simulink model "PMSM_DemoBackup"  (R2020a)
settings: Solver=FixedStepDiscrete  StartTime=0.0  StopTime=Inf  FixedStep=1000e-6  RelTol=1e-3  EnableMultiTasking=on
PreLoadFcn:
  | run('PMSM_Demo_ini.m');
PostLoadFcn:
  | , if any(exist('dsrtsu_mdlpostloadfcn', 'file') ~= 0), dsrtsu_mdlpostloadfcn('Execute', bdroot); end,
InitFcn:
  | , if any(exist('rtifpga_mdlclblib', 'file') ~= 0), rtifpga_mdlclblib('Init', bdroot); end,
undefined symbols (not defined in the file): clock, Const_Id_Fieldweakening, Const_Ld_Stator, Const_Lq_Stator, Const_PolePairs, Const_Psi, Newton, PMSM_Ctrl_Ctrl_mode_SW, PMSM_Ctrl_fRS_Set, PMSM_Ctrl_i_d_Set, PMSM_Ctrl_i_d_Stroke, PMSM_Ctrl_i_q_Set, PMSM_Ctrl_i_q_Stroke, PMSM_Ctrl_Ki_id, PMSM_Ctrl_Ki_iq, PMSM_Ctrl_Ki_n, PMSM_Ctrl_Kp_id, PMSM_Ctrl_Kp_iq, PMSM_Ctrl_Kp_n, PMSM_Ctrl_Limit_iq, PMSM_Ctrl_load_torque, PMSM_Ctrl_n_Limit, PMSM_Ctrl_n_Set, PMSM_Ctrl_n_Stroke, PMSM_Ctrl_Pos_Src, PMSM_Ctrl_TF_Id, PMSM_Ctrl_TF_Iq, PMSM_Ctrl_TF_n, PMSM_Ctrl_theta_offset, PMSM_Ctrl_v_d_Set, PMSM_Ctrl_V_DCLink_Limit, PMSM_Ctrl_v_q_Set, PMSM_Ctrl_Vel_Src, Raphson, rpm_to_rad, s, SW_Fieldweakening, T_PWM
libraries: simulink x37, rti1202lib_adc_class1 x8, dsextras x4, rtiemclib x4, rti1202lib_dio_class1 x3, ASM_ElectricComponents_lib x2, ASM_Utils_lib x1, rti1202lib_base x1
(part 1 of 4)
settings Model: RTICANMMDATA=struct('GeneralSetupData',struct('modelroot','D:\PMSM_ControlDesk','generalsettings',struct('filesettings',struct('destfolder',struct('Name','RTICANMM_FILES','Check',1),'buildfolder',struct('Name','.','Check',1),'AbsDestfolder',struct('Name','D:\PMSM_ControlDesk\RTICANMM_FILES'),'AbsBuildfolder',struct('Name','D:\PMSM_ControlDesk'))),'options',struct('addpaths',1,'rmpaths',1,'addtrcexclusion',true,'cannavigator',struct('checkmonitoring',0),'show_usrtrc',0,'use_usrtrc',0),'advanced',struct('options',ones(1,100)),'MPSetup',{{}},'RTI',struct('Type','RTI1202','Ver','7.15','Date','02-Nov-2020'),'modelname','PMSM_DemoBackup','block','PMSM_DemoBackup'))  RTILINMMDATA=struct('GeneralSetupData',[])  DSRTSU_INTERNAL_RTI_VER=570  DSRTSU_INTERNAL_RTI_TYPE=rti1202  DSRTSU_INTERNAL_RTIFPGA=170  Creator=JesseL  LastModifiedBy=PC2
settings DataIOCC: LimitDataPoints=on  SaveFormat=Array  SignalLoggingSaveFormat=ModelDataLogs  ReturnWorkspaceOutputs=off
settings OptimizationCC: BlockReduction=off  ConditionallyExecuteInputs=off  OptimizeBlockIOStorage=off  BufferReuse=off  GlobalBufferReuse=off  ExpressionFolding=off  ExpressionDepthLimit=2147483647  LocalBlockOutputs=off  InitFltsAndDblsToZero=on  LifeSpan=inf  OptimizeDataStoreBuffers=off  BusAssignmentInplaceUpdate=off
settings DebuggingCC: SaveWithParameterizedLinksMsg=none  UnderspecifiedInitializationDetection=Classic  MergeDetectMultiDrivingBlocksExec=none  SignalResolutionControl=TryResolveAllWithWarning  SolverPrmCheckMsg=warning  MultiTaskDSMMsg=warning  MultiTaskCondExecSysMsg=none  AllowSymbolicDim=off  StateNameClashWarn=warning  SFUnexpectedBacktrackingDiag=warning  SFNoUnconditionalDefaultTransitionDiag=warning  SFExecutionAtInitializationDiag=none  ArithmeticOperatorsInVariantConditions=warning
settings HardwareCC: ProdBitPerPointer=32  ProdBitPerSizeT=32  ProdBitPerPtrDiffT=32  ProdLargestAtomicInteger=Integer  ProdEndianess=BigEndian  ProdWordSize=32  ProdHWDeviceType=Custom Processor->Custom  TargetIntDivRoundTo=Zero  TargetEndianess=BigEndian  TargetHWDeviceType=Custom Processor->Custom
settings ModelReferenceCC: PropagateSignalLabelsOutOfModel=off
settings SFSimCC: SimUseLocalCustomCode=off  MATLABDynamicMemAlloc=off  CustomCodeUndefinedFunction=UseInterfaceOnly
settings RTWCC: Description=dSPACE DS1202 Hardware Platform  SystemTargetFile=rti1202.tlc  MakeCommand=make_rti  TemplateMakefile=rti1202.tmf  RTWUseLocalCustomCode=off
settings CodeAppCC: StateflowObjectComments=on
settings STFCustomTargetCC: ParMdlRefBuildCompliant=on  SystemTargetFile=rti1202.tlc
settings GRTTargetCC: TargetLangStandard=C89/C90 (ANSI)  CompOptLevelCompliant=off  ConcurrentExecutionCompliant=off  CombineOutputUpdateFcns=off  MatFileLogging=off  CPPClassGenCompliant=off  UseToolchainInfoCompliant=off  ExtModeMexFile=noextcomm
settings ConfigComp: CovMetricSettings=dw  CovHtmlReporting=on  CovSaveCumulativeToWorkspaceVar=on  CovSaveSingleToWorkspaceVar=on  CovExternalEMLEnable=off

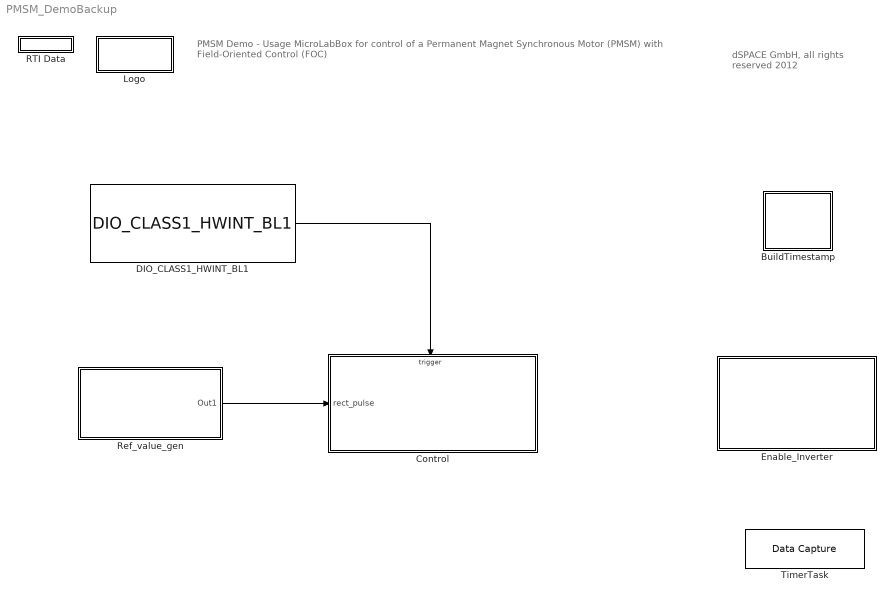
== system PMSM_DemoBackup ==
  note: PMSM Demo - Usage MicroLabBox for control
      | of a Permanent Magnet Synchronous Motor (PMSM)
      | with Field-Oriented Control (FOC)
  note: dSPACE GmbH,
      | all rights reserved 2012
  BuildTimestamp : Subsystem
  Control : Subsystem
  DIO_CLASS1_HWINT_BL1 : rti1202lib_dio_class1/DIO_CLASS1_HWINT_BL1  DSProperties=struct('RTI',struct('Version',uint32(2),'BlockType',struct('isSLSource',uint8(1),'isSLSink',uint8(0),'isHWSource',uint8(0),'isHWSink',uint8(0),'isSetup',uint8(0),'isInline',uint8(1),'isNonInline',uint8(0),'isInterrupt',uint8(1),'isChannelwise',uint8(0)),'IOBoardType',{{'DS120X','STD','DIOC1'}},'UnitType','DSTASKTOOL','Identifier','HWINT','DialogType','ML','BlockSet','NONE','SlaveProcessor','NONE'))  RTIBlockInterface=struct('OutputPortsActive',1,'OutputPortsWidth',int32(1),'OutputPortsName',{{'Interrupt'}},'FunctionCall',uint32(0),'DialogFcn','rti120xstddioc1hwintgui','InitLevel',3,'BlockDisplay',{{['DIO CL1 HWINT\nPort: 1\nChannel: 7'],'center'}},'IconTransparency','on','BlockName',struct('Token',{{'DIO_CLASS1_HWINT_BL1'}}))  RTIBlockParameters=struct('SourceBlockListIdx',{{2,'OFF',[1 2]}},'SourceBlockIdentifier',{{'MCPWM','OFF',[]}},'InterruptTypeListIdx',{{2,'OFF',[1 2]}},'InterruptType',{{['Center position'],'OFF',[]}},'PortNo',{{1,'OFF',[]}},'ChannelNo',{{7,'OFF',[]}})  RTISFcnParameters=struct('PortNo','int16','ChannelNo','int16')  RTIBlockParaDefault=struct('SourceBlockListIdx',1,'SourceBlockIdentifier',['NOT SELECTED'],'InterruptTypeListIdx',1,'InterruptType',['NOT SELECTED'],'PortNo',-1,'ChannelNo',-1)
  Enable_Inverter : Subsystem
      mask Display: disp('Enable_Inverter')
  Logo : Subsystem  mask(dSPACE){EmptyParameter=[]}
      mask prompts: EmptyParameter "Mask Parameter 1:"
      settings: OpenFcn=;
      mask Display: image(imread('rti_mdl_dslogo.tif'));
  RTI Data : Subsystem  Tag=struct('RTIDataServer',struct('RTIDataServerVs','2','RTIModelDescription','struct(''main'',''PMSM_DemoBackup'',''sub'','''',''isMp'',0)'))  LoadFcn="if exist('rtidc'), try,  rtidc('DataHostBlockClbLoad', gcbh); catch, disp(['Warning: ''LoadFcn'' for RTI Data block failed: ' lasterr]); end, end,"  mask(RTI_DATA_HOST){}
      mask help:
      | RTI Data Block.
      | This block is used by RTI to store internal model-dependent data.
      | Please keep this block on the root level of the model. Deleting this block will result in data loss.
      |
      | NEVER DELETE OR COPY THIS BLOCK!
      settings: CopyFcn="if exist('rtidc'), try,  rtidc('DataHostBlockClbCopy', gcbh); catch, disp(['Warning: ''CopyFcn'' for RTI Data block failed: ' lasterr]); end, end,"  DeleteFcn="if exist('rtidc'), try,  rtidc('DataHostBlockClbDelete', gcbh); catch, disp(['Warning: ''DeleteFcn'' for RTI Data block failed: ' lasterr]); end, end,"  ModelCloseFcn="if exist('rtidc'), try,  rtidc('DataHostBlockClbModelClose', gcbh); catch, disp(['Warning: ''ModelCloseFcn'' for RTI Data block failed: ' lasterr]); end, end,"  PreSaveFcn="if exist('rtidc'), try,  rtidc('DataHostBlockClbPreSave', gcbh); catch, disp(['Warning: ''PreSaveFcn'' for RTI Data block failed: ' lasterr]); end, end,"  PostSaveFcn="if exist('rtidc'), try,  rtidc('DataHostBlockClbPostSave', gcbh); catch, disp(['Warning: ''PostSaveFcn'' for RTI Data block failed: ' lasterr]); end, end,"  NameChangeFcn="if exist('rtidc'), try,  rtidc('DataHostBlockClbNameChange', gcbh); catch, disp(['Warning: ''NameChangeFcn'' for RTI Data block failed: ' lasterr]); end, end,"
      mask Help:
      | RTI Data Block.
      | This block is used by RTI to store internal model-dependent data.
      | Please keep this block on the root level of the model. Deleting this block will result in data loss.
      | 
      | NEVER DELETE OR COPY THIS BLOCK!
      mask Display:
      | text(0.5, 0.5, 'RTI Data', 'HorizontalAlignment', 'center');
      | plot([1 0]);
  Ref_value_gen : Subsystem
      mask Display: disp('Generate Reference Values')
  TimerTask : dsextras/Data Capture  ServiceNumber=4  ServiceName=TimerTask_top  SampleTime=-1  XAxisLabelMode=off  XAxisLabel=sec  XAxisIncrement=1  TLCFileName=rti_data_capture  XAxisUnit=[]  IncrementSetting=[]  CustomSampleTime=[]  Reserved1=[]  Reserved2=[]  Reserved3=[]  Reserved4=[]  DSProperties=struct('RTI',struct('Version',uint32(3),'BlockType',struct('isSLSource',uint8(0),'isSLSink',uint8(0),'isHWSource',uint8(0),'isHWSink',uint8(0),'isSetup',uint8(0),'isInline',uint8(1),'isNonInline',uint8(0),'isInterrupt',uint8(0),'isChannelwise',uint8(0)),'IOBoardType','EXTRAS','UnitType','DATACAP','Identifier','DATACAP','DialogType','SL','BlockSet','NONE','SlaveProcessor','NONE'))  RTIBlockInterface=struct('OutputPortsActive',0,'OutputPortsWidth',int32(0),'InitLevel',2,'BlockDisplay',{{['Host Service #4\nTimerTask_top'],'center'}},'BlockName',struct('Token',{{['Data Capture']}}),'MaskDescription',['Places the host service code for ControlDesk in a specific task.'],'IconTransparency','off','SampleTime',{{-1}})  RTIBlockParameters=struct('ServiceNumber',{{4,'OFF',[]}},'ServiceName',{{'TimerTask_top','OFF',[]}},'SampleTime',{{-1,'OFF',[]}},'XAxisLabelMode',{{false,'OFF',[]}},'XAxisLabel',{{'sec','OFF',[]}},'XAxisIncrement',{{1,'OFF',[]}},'TLCFileName',{{'rti_data_capture','OFF',[]}})  RTISFcnParameters=struct('ServiceNumber','double','ServiceName','char','SampleTime','double','XAxisLabelMode','double','XAxisLabel','char','XAxisIncrement','double','TLCFileName','char')  RTIBlockParaDefault=struct('ServiceNumber',1,'ServiceName','ServiceName','SampleTime',-1,'XAxisLabelMode',0,'XAxisLabel','sec','XAxisIncrement',1,'TLCFileName','rti_data_capture')
  wires:
  Ref_value_gen/1(Out1) -> Control/1(rect_pulse)
  DIO_CLASS1_HWINT_BL1/1 -> Control/Trigger

== system PMSM_DemoBackup/BuildTimestamp ==
  Demux : Demux  Outputs=6
  Terminator{,1..5} (6 alike) : Terminator
  clock : Constant  Value=clock()
  wires:
  clock/1 -> Demux/1
  Demux/1 -> Terminator/1  "01_year"
  Demux/2 -> Terminator1/1  "02_month"
  Demux/3 -> Terminator2/1  "03_day"
  Demux/4 -> Terminator3/1  "04_hour"
  Demux/5 -> Terminator4/1  "05_minute"
  Demux/6 -> Terminator5/1  "06_second"

== system PMSM_DemoBackup/Control ==
  rect_pulse : Inport
  function : TriggerPort  TriggerType=function-call  VariantControl=Variant
  Control_load_machine : Subsystem
      mask Display: disp('Load machine Ctrl')
  Controller : Subsystem
  Data Capture : dsextras/Data Capture  ServiceNumber=1  ServiceName=ASYNTask  SampleTime=-1  XAxisLabelMode=off  XAxisLabel=sec  XAxisIncrement=1  TLCFileName=rti_data_capture  XAxisUnit=[]  IncrementSetting=[]  CustomSampleTime=[]  Reserved1=[]  Reserved2=[]  Reserved3=[]  Reserved4=[]  DSProperties=struct('RTI',struct('Version',uint32(3),'BlockType',struct('isSLSource',uint8(0),'isSLSink',uint8(0),'isHWSource',uint8(0),'isHWSink',uint8(0),'isSetup',uint8(0),'isInline',uint8(1),'isNonInline',uint8(0),'isInterrupt',uint8(0),'isChannelwise',uint8(0)),'IOBoardType','EXTRAS','UnitType','DATACAP','Identifier','DATACAP','DialogType','SL','BlockSet','NONE','SlaveProcessor','NONE'))  RTIBlockInterface=struct('OutputPortsActive',0,'OutputPortsWidth',int32(0),'InitLevel',2,'BlockDisplay',{{['Host Service #1\nASYNTask'],'center'}},'BlockName',struct('Token',{{['Data Capture']}}),'MaskDescription',['Places the host service code for ControlDesk in a specific task.'],'IconTransparency','off','SampleTime',{{-1}})  RTIBlockParameters=struct('ServiceNumber',{{1,'OFF',[]}},'ServiceName',{{'ASYNTask','OFF',[]}},'SampleTime',{{-1,'OFF',[]}},'XAxisLabelMode',{{false,'OFF',[]}},'XAxisLabel',{{'sec','OFF',[]}},'XAxisIncrement',{{1,'OFF',[]}},'TLCFileName',{{'rti_data_capture','OFF',[]}})  RTISFcnParameters=struct('ServiceNumber','double','ServiceName','char','SampleTime','double','XAxisLabelMode','double','XAxisLabel','char','XAxisIncrement','double','TLCFileName','char')  RTIBlockParaDefault=struct('ServiceNumber',1,'ServiceName','ServiceName','SampleTime',-1,'XAxisLabelMode',0,'XAxisLabel','sec','XAxisIncrement',1,'TLCFileName','rti_data_capture')
  Data Capture_short : dsextras/Data Capture  ServiceNumber=2  ServiceName=ASYNTask_short  SampleTime=-1  XAxisLabelMode=off  XAxisLabel=sec  XAxisIncrement=1  TLCFileName=rti_data_capture  XAxisUnit=[]  IncrementSetting=[]  CustomSampleTime=[]  Reserved1=[]  Reserved2=[]  Reserved3=[]  Reserved4=[]  DSProperties=struct('RTI',struct('Version',uint32(3),'BlockType',struct('isSLSource',uint8(0),'isSLSink',uint8(0),'isHWSource',uint8(0),'isHWSink',uint8(0),'isSetup',uint8(0),'isInline',uint8(1),'isNonInline',uint8(0),'isInterrupt',uint8(0),'isChannelwise',uint8(0)),'IOBoardType','EXTRAS','UnitType','DATACAP','Identifier','DATACAP','DialogType','SL','BlockSet','NONE','SlaveProcessor','NONE'))  RTIBlockInterface=struct('OutputPortsActive',0,'OutputPortsWidth',int32(0),'InitLevel',2,'BlockDisplay',{{['Host Service #2\nASYNTask_short'],'center'}},'BlockName',struct('Token',{{['Data Capture']}}),'MaskDescription',['Places the host service code for ControlDesk in a specific task.'],'IconTransparency','off','SampleTime',{{-1}})  RTIBlockParameters=struct('ServiceNumber',{{2,'OFF',[]}},'ServiceName',{{'ASYNTask_short','OFF',[]}},'SampleTime',{{-1,'OFF',[]}},'XAxisLabelMode',{{false,'OFF',[]}},'XAxisLabel',{{'sec','OFF',[]}},'XAxisIncrement',{{1,'OFF',[]}},'TLCFileName',{{'rti_data_capture','OFF',[]}})  RTISFcnParameters=struct('ServiceNumber','double','ServiceName','char','SampleTime','double','XAxisLabelMode','double','XAxisLabel','char','XAxisIncrement','double','TLCFileName','char')  RTIBlockParaDefault=struct('ServiceNumber',1,'ServiceName','ServiceName','SampleTime',-1,'XAxisLabelMode',0,'XAxisLabel','sec','XAxisIncrement',1,'TLCFileName','rti_data_capture')
  Input : Subsystem
  Output : Subsystem
  pmsm_ctrl_par_sig : Subsystem
      mask Display: disp('pmsm_ctrl_par_sig');
  wires:
  Controller/2(PWM_Duty[a;b;c]) -> Output/2(PWM_Duty[a,b,c])
  Input/4(n[rpm]) -> Controller/4(n[rpm])
  rect_pulse/1 -> pmsm_ctrl_par_sig/1(rect_pulse)
  Input/5(epsilon[rad]) -> Controller/5(epsilon[rad])
  Input/1(T_Sample [s]) -> Controller/1(T_Sample[s])
  Input/3(i_stator(a,b,c)[A]) -> Controller/3(i_stator[a;b;c][A])
  Controller/1(T_Sample [s]) -> Output/1(T_Sample[s])
  Input/2(V_DCLink[V]) -> Controller/2(V_DCLink[V])

== system PMSM_DemoBackup/Enable_Inverter ==
  DIO_CLASS1_BIT_OUT_BL2 : rti1202lib_dio_class1/DIO_CLASS1_BIT_OUT_BL1  DSProperties=struct('RTI',struct('Version',uint32(1),'BlockType',struct('isSLSource',uint8(0),'isSLSink',uint8(1),'isHWSource',uint8(0),'isHWSink',uint8(1),'isSetup',uint8(0),'isInline',uint8(1),'isNonInline',uint8(0),'isInterrupt',uint8(0),'isChannelwise',uint8(1)),'IOBoardType',{{'DS120X','STD','DIOC1'}},'UnitType','BIT','Identifier','BITOUT','DialogType','ML','BlockSet','NONE','SlaveProcessor','NONE'))  RTIBlockInterface=struct('InputPortsWidth',int32(1),'InputPortsActive',1,'InputPortsDataType',{{'SS_BOOLEAN'}},'InputPortsName',{{'In'}},'BlockDisplay',{{['DIO CL1 BIT OUT\nPort: 1\nChannel: 15\nNumber of channels: 1'],'center\'}},'IconTransparency','on','InitLevel',3,'DialogFcn','rti120xstddioc1bitoutgui','BlockName',struct('Token',{{'DIO_CLASS1_BIT_OUT_BL1'}}))  RTIBlockParameters=struct('PortNo',{{1,'OFF',[]}},'ChannelNo',{{15,'OFF',[]}},'ChannelNumOf',{{1,'OFF',[]}},'HighLevel',{{3,'OFF',[1 3]}},'OutputStateInit',{{zeros(1,16),'OFF',[0 1]}},'OutputStateTerm',{{zeros(1,16),'OFF',[0 1]}},'TerminationMode',{{0,'OFF',[0 1]}},'OutputStateTermValidate',{{0,'OFF',[0 1]}},'OutputStateInitSetAll',{{0,'OFF',[0 1]}},'OutputStateTermSetAll',{{0,'OFF',[0 1]}},'EnableEvent',{{0,'OFF',[0 1]}},'EventMode',{{1,'OFF',[1 3]}},'EventOnFalling',{{1,'OFF',[0 1]}},'EventOnRising',{{0,'OFF',[0 1]}},'EventDelay',{{'0','OFF',[0 1.34]}},'EventRate',{{'1','OFF',[1 256]}},'EventBuildCheck',{{false,'OFF',[]}},'TriggerLine',{{1,'OFF',[1 16]}},'EventChannelNoIdx',{{1,'OFF',[1 16]}},'TLCFileName',{{'rti120xdio_c1_bit_out','OFF',[]}})  RTISFcnParameters=struct('PortNo','int16','ChannelNo','int16','ChannelNumOf','int16','HighLevel','int16','OutputStateInit','int16','OutputStateTerm','int16','TerminationMode','int16','OutputStateTermValidate','int16','EnableEvent','int16','EventMode','int16','EventOnFalling','int16','EventOnRising','int16','EventDelay','double','EventRate','int16','TriggerLine','int16','EventChannelNoIdx','int16','TLCFileName','char')  RTIBlockParaDefault=struct('PortNo',1,'ChannelNo',1,'ChannelNumOf',1,'HighLevel',1,'OutputStateInit',zeros(1,16),'OutputStateTerm',zeros(1,16),'TerminationMode',0,'OutputStateTermValidate',0,'OutputStateInitSetAll',0,'OutputStateTermSetAll',0,'EnableEvent',0,'EventMode',1,'EventOnFalling',1,'EventOnRising',0,'EventDelay',0,'EventRate',1,'EventBuildCheck',0,'TriggerLine',1,'EventChannelNoIdx',1,'TLCFileName','rti120xdio_c1_bit_out')
  Data Type Conversion : DataTypeConversion
  Enable : Constant
  TimerTask : dsextras/Data Capture  ServiceNumber=3  ServiceName=TimerTask  SampleTime=-1  XAxisLabelMode=off  XAxisLabel=sec  XAxisIncrement=1  TLCFileName=rti_data_capture  XAxisUnit=[]  IncrementSetting=[]  CustomSampleTime=[]  Reserved1=[]  Reserved2=[]  Reserved3=[]  Reserved4=[]  DSProperties=struct('RTI',struct('Version',uint32(3),'BlockType',struct('isSLSource',uint8(0),'isSLSink',uint8(0),'isHWSource',uint8(0),'isHWSink',uint8(0),'isSetup',uint8(0),'isInline',uint8(1),'isNonInline',uint8(0),'isInterrupt',uint8(0),'isChannelwise',uint8(0)),'IOBoardType','EXTRAS','UnitType','DATACAP','Identifier','DATACAP','DialogType','SL','BlockSet','NONE','SlaveProcessor','NONE'))  RTIBlockInterface=struct('OutputPortsActive',0,'OutputPortsWidth',int32(0),'InitLevel',2,'BlockDisplay',{{['Host Service #3\nTimerTask'],'center'}},'BlockName',struct('Token',{{['Data Capture']}}),'MaskDescription',['Places the host service code for ControlDesk in a specific task.'],'IconTransparency','off','SampleTime',{{-1}})  RTIBlockParameters=struct('ServiceNumber',{{3,'OFF',[]}},'ServiceName',{{'TimerTask','OFF',[]}},'SampleTime',{{-1,'OFF',[]}},'XAxisLabelMode',{{false,'OFF',[]}},'XAxisLabel',{{'sec','OFF',[]}},'XAxisIncrement',{{1,'OFF',[]}},'TLCFileName',{{'rti_data_capture','OFF',[]}})  RTISFcnParameters=struct('ServiceNumber','double','ServiceName','char','SampleTime','double','XAxisLabelMode','double','XAxisLabel','char','XAxisIncrement','double','TLCFileName','char')  RTIBlockParaDefault=struct('ServiceNumber',1,'ServiceName','ServiceName','SampleTime',-1,'XAxisLabelMode',0,'XAxisLabel','sec','XAxisIncrement',1,'TLCFileName','rti_data_capture')
  wires:
  Enable/1 -> Data Type Conversion/1
  Data Type Conversion/1 -> DIO_CLASS1_BIT_OUT_BL2/1

== system PMSM_DemoBackup/Logo ==
  note: $Revision: 1.5 $
  note: $Date: 2008/08/01 14:14:46GMT+01:00 $
  note: $Workfile: demo1401_smd_io.mdl $

== system PMSM_DemoBackup/RTI Data ==
  RTI Data Store : Subsystem  Tag="struct('private',struct('version',struct('dsVer',uint32(2),'dsVerCreation',uint32(2),'RTI',struct('ver','7.5','type','RTI1202')),'access',struct('type','Model','isPerm',1,'created',['03-Feb-2016 10:56:06'],'modified',['06-May-2024 17:59:05'],'location','')),'public',struct('main',struct('data',[]),'sub',struct('name',{{'PMSM_DemoBackup'}},'data',{{struct('TH',struct('thTaskInfo',struct('taskType',{'TIMER','HWINT','TMRINT','SWINT','GLINT'},'tasksNumOf',{1,1,0,0,0},'srcIds',{{'TIMERA'},{'120XDIOCL1MCPWM_MID_OF_PERIODP1Ch7'},{},{},{}},'taskNames',{{['Timer Task 1']},{'DIO_CLASS1_HWINT_BL1'},{},{},{}})),'th_tc',struct('dataType',{'TASK','TASK'},'taskGroupId',{'',''},'taskGroupList',{{},{}},'taskSchedulingPolicy',{'FCFS','FCFS'},'taskType',{'TIMER','HWINT'},'blkh',{-1,['PMSM_DemoBackup/DIO_CLASS1_HWINT_BL1/Common Hardware' char(10) 'Interrupt Interface']},'srcId',{'TIMERA','120XDIOCL1MCPWM_MID_OF_PERIODP1Ch7'},'srcSgnName',{['Timer A interrupt'],['EMC MCPWM Port 1 Channel 7 Center position']},'srcCpuName',{'',''},'taskName',{['Timer Task 1  [0.001] s'],'DIO_CLASS1_HWINT_BL1'},'taskNameDisplayExt',{'',''},'smplTime',{0.001,0},'smplTimeOffs',{0,0},'hasFixedPriority',{0,0},'priority',{2,1},'hasFixedOvc',{0,0},'ovcType',{1,1},'ovcMax',{1,1}),'tc_th',struct('dataType',{'TASK','TASK'},'taskGroupId',{'',''},'taskGroupList',{{},{}},'taskSchedulingPolicy',{'FCFS','FCFS'},'taskType',{'TIMER','HWINT'},'blkh',{-1,['PMSM_DemoBackup/DIO_CLASS1_HWINT_BL1/Common Hardware' char(10) 'Interrupt Interface']},'srcId',{'TIMERA','120XDIOCL1MCPWM_MID_OF_PERIODP1Ch7'},'srcSgnName',{['Timer A interrupt'],['EMC MCPWM Port 1 Channel 7 Center position']},'srcCpuName',{'',''},'taskName',{['Timer Task 1  [0.001] s'],'DIO_CLASS1_HWINT_BL1'},'taskNameDisplayExt',{'',''},'smplTime',{0.001,0},'smplTimeOffs',{0,0},'hasFixedPriority',{0,0},'priority',{2,1},'hasFixedOvc',{0,0},'ovcType',{1,1},'ovcMax',{1,1}),'FSIValue','0','NISValue','1')}})))"  mask(RTI_DATA_STORE){}
      mask help:
      | RTI Data Store Block. This block is used by RTI to store internal model dependent data. Deleting this block will result in data loss.
      |
      | NEVER DELETE, COPY, OR MODIFY THIS BLOCK!
      mask Help:
      | RTI Data Store Block. This block is used by RTI to store internal model dependent data. Deleting this block will result in data loss.
      | 
      | NEVER DELETE, COPY, OR MODIFY THIS BLOCK!
      mask Display: text(0.5, 0.5, ' ', 'HorizontalAlignment', 'center');

== system PMSM_DemoBackup/Ref_value_gen ==
  Bus Creator : BusCreator  Inputs=6
  Choose_reference_Value_iq : Constant  Value=2
  Choose_reference_Value_n : Constant  Value=2
  Const_ref_iq : Constant  Value=0
  Const_ref_n : Constant  Value=0
  Digital Clock : DigitalClock  SampleTime=1000e-6
  Enabled and Triggered Subsystem : Subsystem  TreatAsAtomicUnit=on
  Gain : Gain
  Multiport Switch : MultiPortSwitch  Inputs=2
  Multiport Switch1 : MultiPortSwitch
  Rate Transition : RateTransition  Deterministic=off
  Sig_gen_iq : SignalGenerator  WaveForm=square  Frequency=0.2
  Sig_gen_n : SignalGenerator  WaveForm=square  Frequency=0.2
  Sine_wave_ref_iq : Sin  SampleTime=0
  Terminator : Terminator
  Out1 : Outport  VectorParamsAs1DForOutWhenUnconnected=off
  wires:
  Sig_gen_n/1 -> Multiport Switch/2, Bus Creator/1, Enabled and Triggered Subsystem/1(n_ref)  "Sig_gen_n"
  Rate Transition/1 -> Out1/1
  Const_ref_n/1 -> Multiport Switch/3
  Choose_reference_Value_n/1 -> Multiport Switch/1, Bus Creator/2  "Choose_ref_value_n"
  Sig_gen_iq/1 -> Multiport Switch1/2
  Const_ref_iq/1 -> Multiport Switch1/3
  Choose_reference_Value_iq/1 -> Multiport Switch1/1, Bus Creator/5  "Choose_ref_value_i"
  Sine_wave_ref_iq/1 -> Multiport Switch1/4
  Bus Creator/1 -> Rate Transition/1  "ref_value"
  Multiport Switch1/1 -> Bus Creator/6  "ref_value_iq"
  Multiport Switch/1 -> Bus Creator/3  "ref_value_n"
  Digital Clock/1 -> Gain/1  "sim_time"
  Gain/1 -> Terminator/1
  Enabled and Triggered Subsystem/1(load_ref) -> Bus Creator/4  "load_machine_ref"

== system PMSM_DemoBackup/Control/Control_load_machine ==
  BrakePeriod : Constant  Value=50e-6
  DIO_CLASS1_PWM_BL1 : rti1202lib_dio_class1/DIO_CLASS1_PWM_BL1  DSProperties=struct('RTI',struct('Version',uint32(1),'BlockType',struct('isSLSource',uint8(0),'isSLSink',uint8(1),'isHWSource',uint8(0),'isHWSink',uint8(1),'isSetup',uint8(0),'isInline',uint8(1),'isNonInline',uint8(0),'isInterrupt',uint8(0),'isChannelwise',uint8(1)),'IOBoardType',{{'DS120X','STD','DIOC1'}},'UnitType','PWM','Identifier','PWM','DialogType','ML','BlockSet','NONE','SlaveProcessor','NONE'))  RTIBlockInterface=struct('InputPortsWidth',int32([1 1]),'InputPortsActive',[1 1],'InputPortsName',{{'Period',['Duty Cycle']}},'BlockDisplay',{{['DIO CL1 PWM\nPort: 1\nChannel: 13'],'center'}},'IconTransparency','on','InitLevel',3,'DialogFcn','rti120xstddioc1pwmgui','BlockName',struct('Token',{{'DIO_CLASS1_PWM_BL1'}}))  RTIBlockParameters=struct('PortNo',{{1,'OFF',[]}},'ChannelNo',{{13,'OFF',[]}},'HighLevel',{{3,'OFF',[1 3]}},'UpdateMode',{{2,'OFF',[1 2]}},'InvertingMode',{{1,'OFF',[1 2]}},'DutyCycleInit',{{'0','OFF',[0 1]}},'DutyCycleTerm',{{'0.5','OFF',[0 1]}},'PeriodInit',{{'5e-05','OFF',[1e-7 1.34]}},'PeriodTerm',{{'5e-05','OFF',[1e-7 1.34]}},'TerminationMode',{{0,'OFF',[0 1]}},'OutputTermValidate',{{0,'OFF',[0 1]}},'OutputTermBuildCheck',{{false,'OFF',[]}},'EnableEvent',{{0,'OFF',[0 1]}},'EventMode',{{1,'OFF',[1 3]}},'EventOnFalling',{{1,'OFF',[0 1]}},'EventOnRising',{{0,'OFF',[0 1]}},'EventDelay',{{'0','OFF',[0 1.34]}},'EventRate',{{'1','OFF',[1 256]}},'EventBuildCheck',{{false,'OFF',[]}},'TriggerLine',{{1,'OFF',[1 16]}},'TLCFileName',{{'rti120xdio_c1_pwm','OFF',[]}})  RTISFcnParameters=struct('PortNo','int16','ChannelNo','int16','HighLevel','int16','UpdateMode','int16','InvertingMode','int16','DutyCycleInit','double','DutyCycleTerm','double','PeriodInit','double','PeriodTerm','double','TerminationMode','int16','OutputTermValidate','int16','EnableEvent','int16','EventMode','int16','EventOnFalling','int16','EventOnRising','int16','EventDelay','double','EventRate','int16','TriggerLine','int16','TLCFileName','char')  RTIBlockParaDefault=struct('PortNo',1,'ChannelNo',1,'HighLevel',1,'UpdateMode',1,'InvertingMode',1,'DutyCycleInit',2^-1,'DutyCycleTerm',2^-1,'PeriodInit',5e-5,'PeriodTerm',5e-5,'TerminationMode',0,'OutputTermValidate',0,'OutputTermBuildCheck',0,'EnableEvent',0,'EventMode',1,'EventOnFalling',1,'EventOnRising',0,'EventDelay',0,'EventRate',1,'EventBuildCheck',0,'TriggerLine',1,'TLCFileName','rti120xdio_c1_pwm')
  Data Type Conversion3 : DataTypeConversion
  Load_enable : Constant  Value=0
  Load_gain : Gain  Gain=0.4
  Product1 : Product  RndMeth=Zero
  Switch : Switch  Threshold=0.5
  Terminator : Terminator
  duty_cycle_2_torque : Subsystem
  load_value_man[Nm] : Constant  Value=0
  manual_Load_control : Constant  Value=0
  torque_2_duty_cycle : Subsystem
  torque_2_duty_cycle1 : Subsystem
  wires:
  Switch/1 -> Product1/1
  manual_Load_control/1 -> Switch/2
  Load_enable/1 -> Product1/2
  duty_cycle_2_torque/1(Out_torque[Nm]) -> Terminator/1  "load[Nm]"
  Product1/1 -> DIO_CLASS1_PWM_BL1/2, duty_cycle_2_torque/1(In_duty_cycle[0..1])
  [TAG_SoftECU_load_machine_ref] -> Load_gain/1
  Data Type Conversion3/1 -> Switch/1
  torque_2_duty_cycle1/1(Out_duty_cycle[0..1]) -> Data Type Conversion3/1
  torque_2_duty_cycle/1(Out_duty_cycle[0..1]) -> Switch/3
  load_value_man[Nm]/1 -> torque_2_duty_cycle/1(In_torque[Nm])
  Load_gain/1 -> torque_2_duty_cycle1/1(In_torque[Nm])
  BrakePeriod/1 -> DIO_CLASS1_PWM_BL1/1

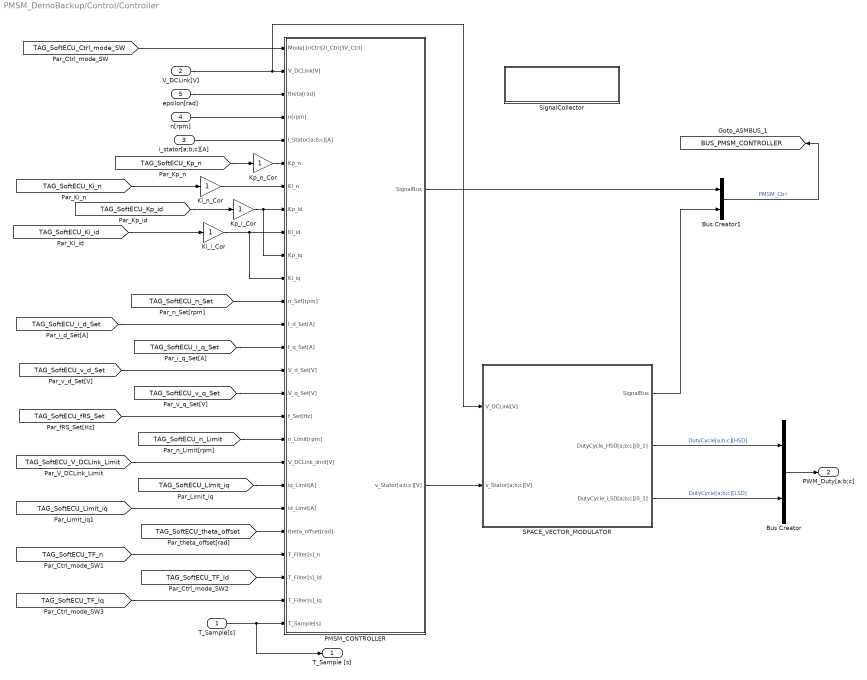
== system PMSM_DemoBackup/Control/Controller ==
  T_Sample[s] : Inport
  V_DCLink[V] : Inport  Port=2
  i_stator[a;b;c][A] : Inport  Port=3
  n[rpm] : Inport  Port=4
  epsilon[rad] : Inport  Port=5
  Bus Creator : BusCreator  Inputs=2
  Bus Creator1 : BusCreator  Inputs=2
  Ki_i_Cor : Gain
  Ki_n_Cor : Gain
  Kp_i_Cor : Gain
  Kp_n_Cor : Gain
  PMSM_CONTROLLER : Subsystem  mask(PSM_CONTROLLER){Const_PolePair=Const_PolePairs, Const_Ld=Const_Ld_Stator, Const_Lq=Const_Lq_Stator, Const_Psi=Const_Psi, Const_Id_Fieldweakening=Const_Id_Fieldweakening, SW_Fieldweakening=SW_Fieldweakening}
      mask prompts: Const_PolePair "Pole pairs []"; Const_Ld "Stator inductance in direct axis Lsd [H]"; Const_Lq "Stator inductance in quadrature axis Lsq [H]"; Const_Psi "Flux induced by magnet Psi[Wb]"; Const_Id_Fieldweakening "Maximum fieldweakening current[A]"; SW_Fieldweakening "Switch fieldweakening mode [1off|2on]"
      mask help: (c) Copyright 2007, dSPACE GmbH. All rights reserved.
      mask Help: eval(['asm_modelhelp(gcbh)'])
  SPACE_VECTOR_MODULATOR : Subsystem  mask(SPACE_VECTOR_MODULATOR){ASMProperties=struct('Name','engine_inertia','Version','1.0','Library','ASM_ElectricComponents_lib')}
      mask help: (c) Copyright 2007, dSPACE GmbH. All rights reserved.
  SignalCollector : Subsystem
  T_Sample [s] : Outport  VectorParamsAs1DForOutWhenUnconnected=off
  PWM_Duty[a;b;c] : Outport  Port=2  VectorParamsAs1DForOutWhenUnconnected=off
  tag scope: BUS_PMSM_CONTROLLER=global
  wires:
  SPACE_VECTOR_MODULATOR/2(DutyCycle_HSD[a;b;c][0_1]) -> Bus Creator/1  "DutyCycle[a;b;c][HSD]"
  SPACE_VECTOR_MODULATOR/3(DutyCycle_LSD[a;b;c][0_1]) -> Bus Creator/2  "DutyCycle[a;b;c][LSD]"
  Bus Creator/1 -> PWM_Duty[a;b;c]/1
  [TAG_SoftECU_v_d_Set] -> PMSM_CONTROLLER/15(V_d_Set[V])
  [TAG_SoftECU_v_q_Set] -> PMSM_CONTROLLER/16(V_q_Set[V])
  [TAG_SoftECU_i_d_Set] -> PMSM_CONTROLLER/13(I_d_Set[A])
  V_DCLink[V]/1 -> PMSM_CONTROLLER/2(V_DCLink[V]), SPACE_VECTOR_MODULATOR/1(V_DCLink[V])
  n[rpm]/1 -> PMSM_CONTROLLER/4(n[rpm])
  i_stator[a;b;c][A]/1 -> PMSM_CONTROLLER/5(i_Stator[a;b;c][A])
  [TAG_SoftECU_fRS_Set] -> PMSM_CONTROLLER/17(f_Set[Hz])
  epsilon[rad]/1 -> PMSM_CONTROLLER/3(theta[rad])
  [TAG_SoftECU_theta_offset] -> PMSM_CONTROLLER/22(theta_offset[rad])
  [TAG_SoftECU_Kp_n] -> Kp_n_Cor/1
  [TAG_SoftECU_Limit_iq] -> PMSM_CONTROLLER/20(iq_Limit[A])
  [TAG_SoftECU_n_Set] -> PMSM_CONTROLLER/12(n_Set[rpm])
  [TAG_SoftECU_n_Limit] -> PMSM_CONTROLLER/18(n_Limit[rpm])
  [TAG_SoftECU_i_q_Set] -> PMSM_CONTROLLER/14(I_q_Set[A])
  [TAG_SoftECU_V_DCLink_Limit] -> PMSM_CONTROLLER/19(V_DCLink_limit[V])
  [TAG_SoftECU_TF_n] -> PMSM_CONTROLLER/23(T_Filter[s]_n)
  [TAG_SoftECU_TF_Id] -> PMSM_CONTROLLER/24(T_Filter[s]_Id)
  PMSM_CONTROLLER/2(v_Stator[a;b;c][V]) -> SPACE_VECTOR_MODULATOR/2(v_Stator[a;b;c][V])
  [TAG_SoftECU_Ki_n] -> Ki_n_Cor/1
  [TAG_SoftECU_Kp_id] -> Kp_i_Cor/1
  [TAG_SoftECU_Ki_id] -> Ki_i_Cor/1
  [TAG_SoftECU_Ctrl_mode_SW] -> PMSM_CONTROLLER/1(Mode[1nCtrl|2I_Ctrl|3V_Ctrl])
  [TAG_SoftECU_TF_Iq] -> PMSM_CONTROLLER/25(T_Filter[s]_Iq)
  T_Sample[s]/1 -> PMSM_CONTROLLER/26(T_Sample[s]), T_Sample [s]/1
  [TAG_SoftECU_Limit_iq] -> PMSM_CONTROLLER/21(id_Limit[A])
  PMSM_CONTROLLER/1(SignalBus) -> Bus Creator1/1
  SPACE_VECTOR_MODULATOR/1(SignalBus) -> Bus Creator1/2
  Bus Creator1/1 -> [BUS_PMSM_CONTROLLER]  "PMSM_Ctrl"
  Kp_n_Cor/1 -> PMSM_CONTROLLER/6(Kp_n)
  Ki_n_Cor/1 -> PMSM_CONTROLLER/7(Ki_n)
  Kp_i_Cor/1 -> PMSM_CONTROLLER/8(Kp_id), PMSM_CONTROLLER/10(Kp_iq)
  Ki_i_Cor/1 -> PMSM_CONTROLLER/9(Ki_id), PMSM_CONTROLLER/11(Ki_iq)

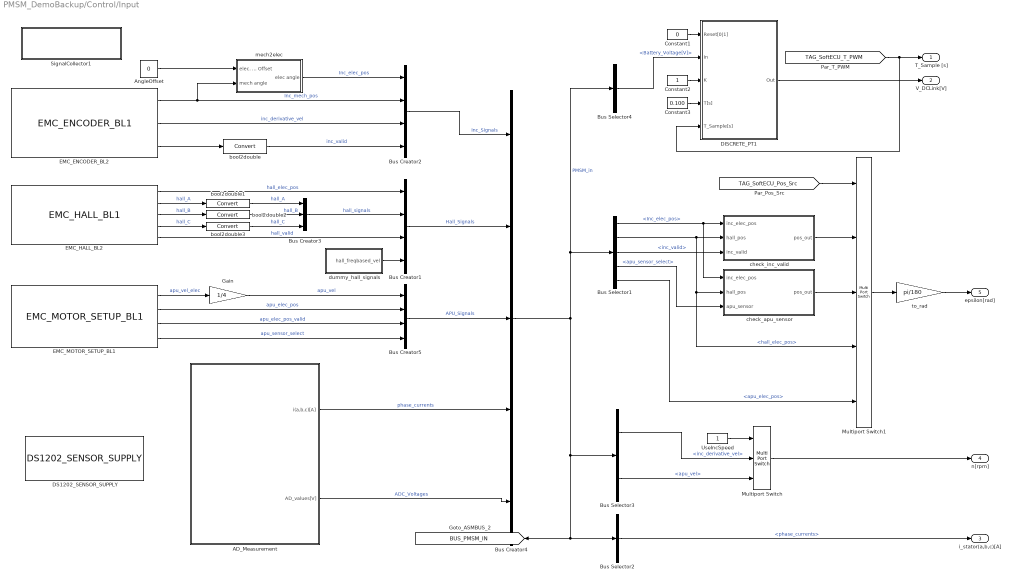
== system PMSM_DemoBackup/Control/Input ==
  AD_Measurement : Subsystem
  AngleOffset : Constant  Value=0
  Bus Creator1 : BusCreator  Inputs=4
  Bus Creator2 : BusCreator  Inputs=4
  Bus Creator3 : BusCreator  Inputs=3
  Bus Creator4 : BusCreator  Inputs=5
  Bus Creator5 : BusCreator  Inputs=4
  Bus Selector1 : BusSelector  OutputSignals=Inc_Signals.Inc_elec_pos,Hall_Signals.hall_elec_pos,Inc_Signals.inc_valid,APU_Signals.apu_sensor_select,APU_Signals.apu_elec_pos
  Bus Selector2 : BusSelector  OutputSignals=phase_currents
  Bus Selector3 : BusSelector  OutputSignals=Inc_Signals.inc_derivative_vel,APU_Signals.apu_vel
  Bus Selector4 : BusSelector  OutputSignals=ADC_Voltages.Battery_Voltage[V]
  Constant1 : Constant  Value=0
  Constant2 : Constant
  Constant3 : Constant  Value=0.100
  DISCRETE_PT1 : Subsystem  mask(DISCRETE_PT1){upper_limit_int=struct('v', 1e300), lower_limit_int=struct('v', -1e300), ASMProperties=struct('Name','DISCRETE_PT1','Version','1.0','Library','ASM_ElectricComponents_lib')}
      mask prompts: upper_limit_int "upper limit (Integrator)"; lower_limit_int "lower limit (Integrator)"
      mask help: (c) Copyright 2007, dSPACE GmbH. All rights reserved.
      mask Help: eval(['asm_modelhelp(gcbh)'])
  DS1202_SENSOR_SUPPLY : rti1202lib_base/DS1202_SENSOR_SUPPLY  DSProperties=struct('RTI',struct('Version',uint32(1),'BlockType',struct('isSLSource',uint8(0),'isSLSink',uint8(0),'isHWSource',uint8(0),'isHWSink',uint8(1),'isSetup',uint8(0),'isInline',uint8(1),'isNonInline',uint8(0),'isInterrupt',uint8(0),'isChannelwise',uint8(0)),'IOBoardType',{{'DS120X','BASE'}},'UnitType','SENSORSUPPLY','Identifier','SENSORSUPPLY','DialogType','ML','BlockSet','NONE','SlaveProcessor','NONE'))  RTIBlockInterface=struct('OutputPortsActive',0,'OutputPortsWidth',int32(0),'DialogFcn','rti120xbasesensorsupplygui','InitLevel',3,'IconTransparency','off','BlockDisplay',{{['DS1202\nSensor Supply'],'center'}},'BlockName',struct('Token',{{'DS1202_SENSOR_SUPPLY'}}))  RTIBlockParameters=struct('Voltage',{{'5','OFF',[2 20]}},'TLCFileName',{{'rti120xbase_sensor_supply','OFF',[]}})  RTISFcnParameters=struct('Voltage','int16','TLCFileName','char')  RTIBlockParaDefault=struct('Voltage',2,'TLCFileName','rti120xbase_sensor_supply')
  EMC_ENCODER_BL2 : rtiemclib/EMC_ENCODER_BL1  DSProperties=struct('RTI',struct('Version',uint32(2),'BlockType',struct('isSLSource',uint8(1),'isSLSink',uint8(0),'isHWSource',uint8(1),'isHWSink',uint8(0),'isSetup',uint8(0),'isInline',uint8(1),'isNonInline',uint8(0),'isInterrupt',uint8(0),'isChannelwise',uint8(1)),'IOBoardType','DSEMC','UnitType','ENCODER','Identifier','ENCODER','DialogType','ML','BlockSet','RTIEMC','SlaveProcessor','NONE'))  RTIBlockInterface=struct('OutputPortsWidth',int32([1 1 1 1 1]),'OutputPortsActive',int32([1 1 1]),'OutputPortsName',{{'Position','Speed','Angle',['Angular Velocity'],['Index Detected']}},'OutputPortsDataType',{{'SS_DOUBLE','SS_DOUBLE','SS_DOUBLE','SS_DOUBLE','SS_BOOLEAN'}},'InitLevel',3,'IconTransparency','on','BlockDisplay',{{['EMC Encoder\nUnit: 1\nDIO class: 1\nPort: 1\nChannel: 4'],'center'}},'DialogFcn','rtiemcencodergui','BlockName',struct('Token',{{'EMC_ENCODER_BL1'}}))  RTIBlockParameters=struct('UnitNo',{{1,'OFF',[1 6]}},'DioClassNo',{{1,'OFF',[1 2]}},'PortNo',{{1,'OFF',[1 3]}},'ChannelNo',{{4,'OFF',[1 14]}},'HwSignalPin',{{['DIO1 ch1'],'OFF',[]}},'HwRefPin',{{'GND','OFF',[]}},'EnablePosMeasurement',{{0,'OFF',[0 1]}},'IndexSetMode',{{3,'OFF',[1 3]}},'NumOfLines',{{'2500','OFF',[1 2097152]}},'InitAngleValue',{{'353','OFF',[0 359.99999]}},'IndexAngleValue',{{'353','OFF',[0 359.99999]}},'MinPosValue',{{'-2097152','OFF',[-2097152 2097150.75]}},'MaxPosValue',{{'2097151.75','OFF',[-2097151 2097151.75]}},'InitPosValue',{{'0','OFF',[-2097152 2097151.75]}},'IndexPosValue',{{'0','OFF',[-2097152 2097151.75]}},'IndexGateMode',{{1,'OFF',[0 1]}},'EnableNoiseFilter',{{0,'OFF',[0 1]}},'FilterInterval',{{'0','OFF',[0 0.01]}},'IndexDetectedOutPortMode',{{1,'OFF',[0 1]}},'BuildCheckAngleMeasurement',{{1,'OFF',[0 1]}},'BuildCheckAngleIndexMode',{{1,'OFF',[0 1]}},'BuildCheckPosIndexMode',{{0,'OFF',[0 1]}},'TLCFileName',{{'rtiemcencoder','OFF',[]}},'EnableMinSpeed',{{0,'OFF',[0 1]}},'MinSpeedAngleValue',{{45,'OFF',[0.01 10000]}},'MinSpeedPosValue',{{100,'OFF',[1 1000000]}},'BuildCheckAngleMinSpeed',{{0,'OFF',[0 1]}},'BuildCheckPosMinSpeed',{{0,'OFF',[0 1]}})  RTISFcnParameters=struct('UnitNo','int32','DioClassNo','int32','PortNo','int32','ChannelNo','int32','EnablePosMeasurement','int32','IndexSetMode','int32','IndexDetectedOutPortMode','int32','NumOfLines','uint32','InitAngleValue','double','IndexAngleValue','double','MinPosValue','double','MaxPosValue','double','InitPosValue','double','IndexPosValue','double','IndexGateMode','int32','EnableNoiseFilter','int32','FilterInterval','double','TLCFileName','char','EnableMinSpeed','int32','MinSpeedAngleValue','double','MinSpeedPosValue','double')  RTIBlockParaDefault=struct('UnitNo',1,'DioClassNo',1,'PortNo',1,'ChannelNo',1,'HwSignalPin',['DIO1 ch1'],'HwRefPin','GND','EnablePosMeasurement',0,'IndexSetMode',1,'NumOfLines',1024,'InitAngleValue',60,'IndexAngleValue',0,'MinPosValue',-2097152,'MaxPosValue',2097151.75,'InitPosValue',0,'IndexPosValue',0,'IndexGateMode',0,'EnableNoiseFilter',0,'FilterInterval',0,'IndexDetectedOutPortMode',0,'BuildCheckAngleMeasurement',0,'BuildCheckAngleIndexMode',0,'BuildCheckPosIndexMode',0,'TLCFileName','rtiemcencoder','EnableMinSpeed',0,'MinSpeedAngleValue',45,'MinSpeedPosValue',100,'BuildCheckAngleMinSpeed',0,'BuildCheckPosMinSpeed',0)
      settings: SourceProductName=dSPACE RTI Electric Motor Control Blockset
  EMC_HALL_BL2 : rtiemclib/EMC_HALL_BL1  DSProperties=struct('RTI',struct('Version',uint32(1),'BlockType',struct('isSLSource',uint8(1),'isSLSink',uint8(0),'isHWSource',uint8(1),'isHWSink',uint8(0),'isSetup',uint8(0),'isInline',uint8(1),'isNonInline',uint8(0),'isInterrupt',uint8(0),'isChannelwise',uint8(0)),'IOBoardType','DSEMC','UnitType','HALL','Identifier','HALL','DialogType','ML','BlockSet','RTIEMC','SlaveProcessor','NONE'))  RTIBlockInterface=struct('InputPortsWidth',int32(1),'InputPortsActive',0,'InputPortsName',{{'Offset'}},'OutputPortsWidth',int32([1 1 1 1 1]),'OutputPortsActive',[1 1 1 1 1],'OutputPortsDataType',{{'SS_DOUBLE','SS_BOOLEAN','SS_BOOLEAN','SS_BOOLEAN','SS_BOOLEAN'}},'OutputPortsName',{{'Position',['Signal A'],['Signal B'],['Signal C'],['Signal Valid']}},'BlockDisplay',{{['EMC Hall\nUnit: 1\nDIO Class: 1\nPort: 1\nChannel: 1'],'center'}},'IconTransparency','on','InitLevel',3,'DialogFcn','rtiemchallgui','BlockName',struct('Token',{{'EMC_HALL_BL1'}}))  RTIBlockParameters=struct('UnitNo',{{1,'OFF',[1 2]}},'DioClassNo',{{1,'OFF',[1 2]}},'PortNo',{{1,'OFF',[1 3]}},'ChannelNo',{{1,'OFF',[1 14]}},'SensorARisingEdge',{{'353','OFF',[0 359.999]}},'SensorAFallingEdge',{{'173','OFF',[0 359.999]}},'SensorBRisingEdge',{{'113','OFF',[0 359.999]}},'SensorBFallingEdge',{{'293','OFF',[0 359.999]}},'SensorCRisingEdge',{{'233','OFF',[0 359.999]}},'SensorCFallingEdge',{{'53','OFF',[0 359.999]}},'PositionOffset',{{'0','OFF',[-60 60]}},'EnableSensorsOffsetPort',{{0,'OFF',[0 1]}},'ReverseDirection',{{0,'OFF',[0 1]}},'EnableSignalPorts',{{1,'OFF',[0 1]}},'EnableSignalsValidPort',{{1,'OFF',[0 1]}},'EnableNoiseFilter',{{0,'OFF',[0 1]}},'FilterInterval',{{'0','OFF',[0 0.01]}},'TLCFileName',{{'rtiemchall','OFF',[]}})  RTISFcnParameters=struct('UnitNo','int32','DioClassNo','int32','PortNo','int32','ChannelNo','int32','SensorARisingEdge','double','SensorAFallingEdge','double','SensorBRisingEdge','double','SensorBFallingEdge','double','SensorCRisingEdge','double','SensorCFallingEdge','double','PositionOffset','double','EnableSensorsOffsetPort','int32','ReverseDirection','int32','EnableSignalPorts','int32','EnableSignalsValidPort','int32','EnableNoiseFilter','int32','FilterInterval','double','TLCFileName','char')  RTIBlockParaDefault=struct('UnitNo',1,'DioClassNo',1,'PortNo',1,'ChannelNo',1,'SensorARisingEdge',0,'SensorAFallingEdge',180,'SensorBRisingEdge',120,'SensorBFallingEdge',300,'SensorCRisingEdge',240,'SensorCFallingEdge',60,'PositionOffset',0,'EnableSensorsOffsetPort',0,'ReverseDirection',0,'EnableSignalPorts',0,'EnableSignalsValidPort',0,'EnableNoiseFilter',0,'FilterInterval',0,'TLCFileName','rtiemchall')
      settings: SourceProductName=dSPACE RTI Electric Motor Control Blockset
  EMC_MOTOR_SETUP_BL1 : rtiemclib/EMC_MOTOR_SETUP_BL1  DSProperties=struct('RTI',struct('Version',uint32(1),'BlockType',struct('isSLSource',uint8(1),'isSLSink',uint8(0),'isHWSource',uint8(1),'isHWSink',uint8(0),'isSetup',uint8(1),'isInline',uint8(1),'isNonInline',uint8(0),'isInterrupt',uint8(0),'isChannelwise',uint8(1)),'IOBoardType','DSEMC','UnitType','MOTORSETUP','Identifier','MOTORSETUP','DialogType','ML','BlockSet','RTIEMC','SlaveProcessor','NONE'))  RTIBlockInterface=struct('OutputPortsWidth',int32([1 1 1 1 1 1]),'OutputPortsActive',[1 1 1 0 0 1],'OutputPortsDataType',{{'SS_DOUBLE','SS_DOUBLE','SS_BOOLEAN','SS_DOUBLE','SS_BOOLEAN','SS_UINT32'}},'OutputPortsName',{{'Speed',['Electr. Position'],['Electr. Position Valid'],['Mech. Position'],['Mech. Position Valid'],'Sensor'}},'BlockDisplay',{{['EMC Motor Setup\nUnit: 1'],'center'}},'IconTransparency','on','InitLevel',3,'DialogFcn','rtiemcmotorsetupgui','BlockName',struct('Token',{{'EMC_MOTOR_SETUP_BL1'}}))  RTIBlockParameters=struct('UnitNo',{{1,'OFF',[1 4]}},'SensorA_Idx',{{2,'OFF',[1 2]}},'SensorA_TypeNo',{{1,'OFF',[]}},'SensorA_UnitNo',{{1,'OFF',[]}},'SensorA_ClassNo',{{1,'OFF',[]}},'SensorA_PortNo',{{1,'OFF',[]}},'SensorA_ChannelNo',{{1,'OFF',[]}},'SensorA_PolePairs',{{4,'OFF',[]}},'SensorB_Idx',{{2,'OFF',[1 2]}},'SensorB_TypeNo',{{1,'OFF',[]}},'SensorB_UnitNo',{{1,'OFF',[]}},'SensorB_ClassNo',{{1,'OFF',[]}},'SensorB_PortNo',{{1,'OFF',[]}},'SensorB_ChannelNo',{{4,'OFF',[]}},'Actor_Idx',{{1,'OFF',1}},'Actor_TypeNo',{{1,'OFF',[]}},'Actor_UnitNo',{{-1,'OFF',[]}},'Actor_ClassNo',{{-1,'OFF',[]}},'Actor_PortNo',{{-1,'OFF',[]}},'Actor_ChannelNo',{{-1,'OFF',[]}},'Actor_PolePairs',{{4,'OFF',[]}},'EnablePortMechPos',{{0,'OFF',[0 1]}},'EnablePortSensor',{{1,'OFF',[0 1]}},'EnableEvent',{{0,'OFF',[0 1]}},'EventMode',{{1,'OFF',[1 3]}},'EventBasedOnSensorIdx',{{1,'OFF',[1 3]}},'EventBasedOnSensor',{{['NOT SELECTED'],'OFF',[]}},'EventBasedOnAngle',{{1,'OFF',[1 2]}},'EnablePeriodicInterrupt',{{1,'OFF',[0 1]}},'EnablePos1Interrupt',{{0,'OFF',[0 1]}},'EnablePos2Interrupt',{{0,'OFF',[0 1]}},'EnablePos3Interrupt',{{0,'OFF',[0 1]}},'EnablePos4Interrupt',{{0,'OFF',[0 1]}},'AngleInterval',{{'1','OFF',[1.34e-6 360]}},'StartAngle',{{'0','OFF',[0 0.99999866]}},'AngleBuildCheck',{{false,'OFF',[]}},'TriggerSource',{{1,'OFF',[1 6]}},'TriggerLine',{{1,'OFF',[1 16]}},'TLCFileName',{{'rtiemcmotorsetup','OFF',[]}})  RTISFcnParameters=struct('UnitNo','int32','SensorA_Idx','int32','SensorA_TypeNo','int32','SensorA_UnitNo','int32','SensorA_PolePairs','int32','SensorB_Idx','int32','SensorB_TypeNo','int32','SensorB_UnitNo','int32','Actor_PolePairs','int32','EnablePortMechPos','int32','EnablePortSensor','int32','EnableEvent','int32','EventMode','int32','EventBasedOnSensorIdx','int32','EventBasedOnAngle','int32','EnablePeriodicInterrupt','int32','EnablePos1Interrupt','int32','EnablePos2Interrupt','int32','EnablePos3Interrupt','int32','EnablePos4Interrupt','int32','AngleInterval','double','StartAngle','double','TriggerSource','int32','TriggerLine','int32','TLCFileName','char')  RTIBlockParaDefault=struct('UnitNo',1,'SensorA_Idx',1,'SensorA_TypeNo',1,'SensorA_UnitNo',-1,'SensorA_ClassNo',-1,'SensorA_PortNo',-1,'SensorA_ChannelNo',-1,'SensorA_PolePairs',1,'SensorB_Idx',1,'SensorB_TypeNo',1,'SensorB_UnitNo',-1,'SensorB_ClassNo',-1,'SensorB_PortNo',-1,'SensorB_ChannelNo',-1,'Actor_Idx',1,'Actor_TypeNo',1,'Actor_UnitNo',-1,'Actor_ClassNo',-1,'Actor_PortNo',-1,'Actor_ChannelNo',-1,'Actor_PolePairs',1,'EnablePortMechPos',0,'EnablePortSensor',0,'EnableEvent',0,'EventMode',1,'EventBasedOnSensorIdx',1,'EventBasedOnSensor',['NOT SELECTED'],'EventBasedOnAngle',1,'EnablePeriodicInterrupt',1,'EnablePos1Interrupt',0,'EnablePos2Interrupt',0,'EnablePos3Interrupt',0,'EnablePos4Interrupt',0,'AngleInterval',1,'StartAngle',0,'AngleBuildCheck',0,'TriggerSource',1,'TriggerLine',1,'TLCFileName','rtiemcmotorsetup')
      settings: SourceProductName=dSPACE RTI Electric Motor Control Blockset
  Gain : Gain  Gain=1/4
  Multiport Switch : MultiPortSwitch  Inputs=2
  Multiport Switch1 : MultiPortSwitch  Inputs=4
  SignalCollector1 : Subsystem
  UseIncSpeed : Constant
  bool2double{,1..3} (4 alike) : DataTypeConversion
  check_apu_sensor : Subsystem
  check_inc_valid : Subsystem
  dummy_hall_signals : Subsystem
  mech2elec : Subsystem
  to_rad : Gain  Gain=pi/180
  T_Sample [s] : Outport  VectorParamsAs1DForOutWhenUnconnected=off
  V_DCLink[V] : Outport  Port=2  VectorParamsAs1DForOutWhenUnconnected=off
  i_stator(a,b,c)[A] : Outport  Port=3  VectorParamsAs1DForOutWhenUnconnected=off
  n[rpm] : Outport  Port=4  VectorParamsAs1DForOutWhenUnconnected=off
  epsilon[rad] : Outport  Port=5  VectorParamsAs1DForOutWhenUnconnected=off
  tag scope: BUS_PMSM_IN=global
  wires:
  Multiport Switch1/1 -> to_rad/1
  [TAG_SoftECU_Pos_Src] -> Multiport Switch1/1
  [TAG_SoftECU_T_PWM] -> T_Sample [s]/1, DISCRETE_PT1/5(T_Sample[s])
  AD_Measurement/1(i(a,b,c)[A]) -> Bus Creator4/4  "phase_currents"
  AD_Measurement/2(AD_values[V]) -> Bus Creator4/5  "ADC_Voltages"
  Bus Selector2/1 -> i_stator(a,b,c)[A]/1  "<phase_currents>"
  Bus Selector1/1 -> check_inc_valid/1(inc_elec_pos), check_apu_sensor/1(inc_elec_pos)  "<Inc_elec_pos>"
  Bus Selector1/2 -> check_inc_valid/2(hall_pos), Multiport Switch1/4, check_apu_sensor/2(hall_pos)  "<hall_elec_pos>"
  Bus Selector1/3 -> check_inc_valid/3(inc_valid)  "<inc_valid>"
  check_inc_valid/1(pos_out) -> Multiport Switch1/2
  Bus Selector4/1 -> DISCRETE_PT1/2(In)  "<Battery_Voltage[V]>"
  Constant1/1 -> DISCRETE_PT1/1(Reset[0|1])
  Constant2/1 -> DISCRETE_PT1/3(K)
  Constant3/1 -> DISCRETE_PT1/4(T[s])
  DISCRETE_PT1/1(Out) -> V_DCLink[V]/1
  Bus Creator2/1 -> Bus Creator4/1  "Inc_Signals"
  EMC_ENCODER_BL2/2 -> Bus Creator2/3  "inc_derivative_vel"
  AngleOffset/1 -> mech2elec/1(elec. Angle Offset)
  EMC_ENCODER_BL2/1 -> Bus Creator2/2, mech2elec/2(mech angle)  "Inc_mech_pos"
  mech2elec/1(elec angle) -> Bus Creator2/1  "Inc_elec_pos"
  bool2double/1 -> Bus Creator2/4  "inc_valid"
  EMC_ENCODER_BL2/3 -> bool2double/1
  Bus Creator3/1 -> Bus Creator1/2  "hall_signals"
  Bus Creator1/1 -> Bus Creator4/2  "Hall_Signals"
  EMC_HALL_BL2/1 -> Bus Creator1/1  "hall_elec_pos"
  EMC_HALL_BL2/2 -> bool2double1/1  "hall_A"
  EMC_HALL_BL2/3 -> bool2double2/1  "hall_B"
  EMC_HALL_BL2/4 -> bool2double3/1  "hall_C"
  EMC_HALL_BL2/5 -> Bus Creator1/3  "hall_valid"
  dummy_hall_signals/1(hall_freqbased_vel) -> Bus Creator1/4
  bool2double1/1 -> Bus Creator3/1  "hall_A"
  bool2double2/1 -> Bus Creator3/2  "hall_B"
  bool2double3/1 -> Bus Creator3/3  "hall_C"
  Bus Creator5/1 -> Bus Creator4/3  "APU_Signals"
  EMC_MOTOR_SETUP_BL1/1 -> Gain/1  "apu_vel_elec"
  EMC_MOTOR_SETUP_BL1/2 -> Bus Creator5/2  "apu_elec_pos"
  EMC_MOTOR_SETUP_BL1/3 -> Bus Creator5/3  "apu_elec_pos_valid"
  EMC_MOTOR_SETUP_BL1/4 -> Bus Creator5/4  "apu_sensor_select"
  Gain/1 -> Bus Creator5/1  "apu_vel"
  to_rad/1 -> epsilon[rad]/1
  Bus Selector3/1 -> Multiport Switch/2  "<inc_derivative_vel>"
  Multiport Switch/1 -> n[rpm]/1
  Bus Selector3/2 -> Multiport Switch/3  "<apu_vel>"
  Bus Creator4/1 -> Bus Selector2/1, [BUS_PMSM_IN], Bus Selector3/1, Bus Selector4/1, Bus Selector1/1  "PMSM_in"
  Bus Selector1/4 -> check_apu_sensor/3(apu_sensor)  "<apu_sensor_select>"
  check_apu_sensor/1(pos_out) -> Multiport Switch1/3
  Bus Selector1/5 -> Multiport Switch1/5  "<apu_elec_pos>"
  UseIncSpeed/1 -> Multiport Switch/1
